simulink model "statetest"  (R2015a)
settings: Solver=FixedStepDiscrete  StartTime=0.0  StopTime=10.0  FixedStep=0.01  RelTol=1e-3
settings Model: Creator=Keshav  LastModifiedBy=Keshav

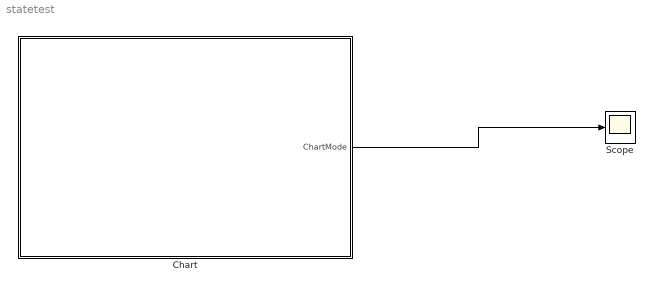
== system statetest ==
  Chart : Stateflow chart  TreatAsAtomicUnit=on
  Scope : Scope
  wires:
  Chart/1(ChartMode) -> Scope/1

== stateflow chart statetest/Chart ==
  state State1
  state State3
  state State2
  (default) -> State1
  State1 -> State2 : after(2, sec)
  State2 -> State3 : after(3, sec)
  data: ChartMode output Enum: ChartModeType
